simulink model "TP_3tanks_sim"  (R2024b)
settings: Solver=FixedStepAuto  StartTime=0.0  StopTime=100  RelTol=1e-3
values from neighbouring files (symbols this model uses):
  g = 9.8    [inverted_script.m]    (also in tanks_variable.m = 9.82)
  k1 = 0.32    [tanks_variable.m]
  k2 = 0.24    [tanks_variable.m]
  mu13 = 3.21    [tanks_variable.m]
  mu20 = 3.21    [tanks_variable.m]
  mu32 = 3.21    [tanks_variable.m]
  S1 = 0.04    [tanks_variable.m]
  S2 = 0.037    [tanks_variable.m]
  S3 = 0.049    [tanks_variable.m]
  Sp = 4e-4    (= 0.0004)    [tanks_variable.m]
libraries: slpidlib x2
settings Model: Creator=thomas  LastModifiedBy=thomas
settings OptimizationCC: DefaultParameterBehavior=Inlined  EnhancedBackFolding=on  PassReuseOutputArgsAs=Individual arguments  ZeroExternalMemoryAtStartup=off  ZeroInternalMemoryAtStartup=off  MaxStackSize=64  OptimizeBlockOrder=speed  DifferentSizesBufferReuse=on  OptimizationCustomize=off  EfficientTunableParamExpr=on
settings DebuggingCC: ParameterTunabilityLossMsg=error
settings HardwareCC: ProdBitPerLong=64  ProdHWDeviceType=Intel->x86-64 (Linux 64)  UseEmbeddedCoderFeatures=off
settings SFSimCC: MATLABDynamicMemAlloc=off
settings RTWCC: Description=Embedded Coder  SystemTargetFile=ert.tlc  HardwareBoard=Robot Operating System 2 (ROS 2)  TLCOptions="-aInlineSetEventsForThisBaseRateFcn=TLC_FALSE -aSuppressMultiTaskScheduler=TLC_FALSE  -aRateBasedStepFcn=0"  TemplateMakefile=ert_default_tmf  Toolchain=Colcon Tools  TargetLang=C++
settings CodeAppCC: ForceParamTrailComments=on  IgnoreCustomStorageClasses=off  OperatorAnnotations=on  SimulinkDataObjDesc=on  SFDataObjDesc=on  InsertBlockDesc=on
settings ERTTargetCC: CodeInterfacePackaging=C++ class  SupportNonInlinedSFcns=on  RootIOFormat=Structure reference

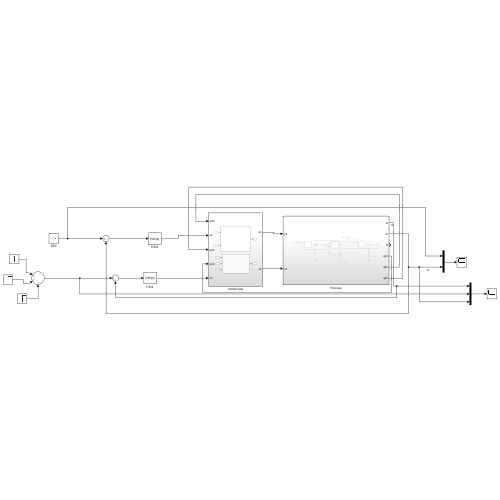
[thumbnail: Simulink's stored preview of the top-level diagram]
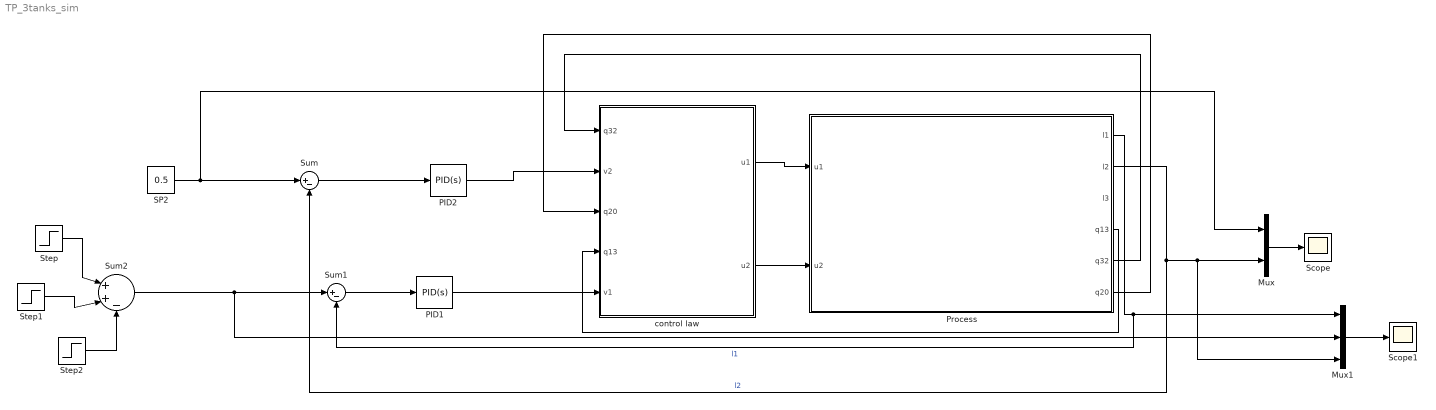
== system TP_3tanks_sim ==
  Mux : Mux  Inputs=2
  Mux1 : Mux  Inputs=3
  PID1 : slpidlib/PID Controller  Controller=PID  Form=Parallel  TimeDomain=Continuous-time  UseExternalTs=off  SampleTime=-1  IntegratorMethod=Forward Euler  FilterMethod=Forward Euler  ControllerParametersSource=internal  P=1  I=1  UseKiTs=off  D=0  UseExternalDerivativeSource=off  N=100  UseFilter=on  TunerSelectOption=Transfer Function Based (PID Tuner App)  InitialConditionSource=internal  InitialConditionForIntegrator=0  InitialConditionForFilter=0  DifferentiatorICPrevScaledInput=0  ExternalReset=none  TrackingMode=off  Kt=1  LimitOutput=off  SatLimitsSource=internal  UpperSaturationLimit=inf  LowerSaturationLimit=-inf  LinearizeAsGain=on  AntiWindupMode=none  Kb=1  LimitIntegrator=off  UpperIntegratorSaturationLimit=inf  LowerIntegratorSaturationLimit=-inf  POutMin=[]  POutMax=[]  IOutMin=[]  IOutMax=[]  DOutMin=[]  DOutMax=[]  NOutMin=[]  NOutMax=[]  SumOutMin=[]  SumOutMax=[]  SaturationOutMin=[]  SaturationOutMax=[]  PParamMin=[]  PParamMax=[]  IParamMin=[]  IParamMax=[]  DParamMin=[]  DParamMax=[]  NParamMin=[]  NParamMax=[]  KbParamMin=[]  KbParamMax=[]  KtParamMin=[]  KtParamMax=[]  KbOutMin=[]  KbOutMax=[]  KtOutMin=[]  KtOutMax=[]  IntegratorOutMin=[]  IntegratorOutMax=[]  FilterOutMin=[]  FilterOutMax=[]  SumI1OutMin=[]  SumI1OutMax=[]  SumI2OutMin=[]  SumI2OutMax=[]  SumI3OutMin=[]  SumI3OutMax=[]  SumI4OutMin=[]  SumI4OutMax=[]  SumDOutMin=[]  SumDOutMax=[]  DifferentiatorOutMin=[]  DifferentiatorOutMax=[]  FilterDiffOutCoefMin=[]  FilterDiffOutCoefMax=[]  ReciprocalOutMin=[]  ReciprocalOutMax=[]  SumDenOutMin=[]  SumDenOutMax=[]  SumNumOutMin=[]  SumNumOutMax=[]  DivideOutMin=[]  DivideOutMax=[]  UdiffTsProdOutMin=[]  UdiffTsProdOutMax=[]  NTsProdOutMin=[]  NTsProdOutMax=[]  UintegralTsProdOutMin=[]  UintegralTsProdOutMax=[]  UngainTsProdOutMin=[]  UngainTsProdOutMax=[]  ClampingZeroOutDataTypeStr=Inherit: Inherit via back propagation  ClampingZeroOutMin=[]  ClampingZeroOutMax=[]  FilterDenConstantOutDataTypeStr=Inherit: Inherit via back propagation  FilterDenConstantOutMin=[]  FilterDenConstantOutMax=[]  PCopyOutDataTypeStr=Inherit: Inherit via back propagation  PCopyOutMin=[]  PCopyOutMax=[]  NCopyOutDataTypeStr=Inherit: Inherit via back propagation  NCopyOutMin=[]  NCopyOutMax=[]  IntegratorContinuousStateAttributes=''  IntegratorStateMustResolveToSignalObject=off  IntegratorRTWStateStorageClass=Auto  FilterContinuousStateAttributes=''  FilterStateMustResolveToSignalObject=off  FilterRTWStateStorageClass=Auto  ParallelPVariant=InternalParameters  IdealPVariant=Disabled  IVariant=InternalParameters  DVariant=InternalParameters  IntegratorVariant=Continuous  SatVariant=Disabled  AWVariant=Passthrough  PCopyVariant=Disabled  TRVariant=Disabled  FdbkBlocksVariant=Forward  IdealPFdbkVariant=Disabled  SatFdbkVariant=Disabled  DerivativeFilterVariant=ContFilter  NVariant=InternalParameters  NCopyVariant=Disabled  FilterICVariant=InternalICsFilter  IntegratorICVariant=InternalICs  ExternalResetVariant=Disabled  TRSumVariant=Passthrough  SumFdbkVariant=Disabled  SumVariant=Sum_PID  TsampFilterVariant=InternalTs  TsampNgainVariant=Passthrough  TsampIntegralVariant=Disabled_SignalSpec  ExternalSaturationOutDataTypeStr=Inherit: Same as second input  DerivativeSourceVariant=ErrorSignal  PreIntVariant=InternalPreInt
  PID2 : slpidlib/PID Controller  Controller=PID  Form=Parallel  TimeDomain=Continuous-time  UseExternalTs=off  SampleTime=-1  IntegratorMethod=Forward Euler  FilterMethod=Forward Euler  ControllerParametersSource=internal  P=1  I=1  UseKiTs=off  D=0  UseExternalDerivativeSource=off  N=100  UseFilter=on  TunerSelectOption=Transfer Function Based (PID Tuner App)  InitialConditionSource=internal  InitialConditionForIntegrator=0  InitialConditionForFilter=0  DifferentiatorICPrevScaledInput=0  ExternalReset=none  TrackingMode=off  Kt=1  LimitOutput=off  SatLimitsSource=internal  UpperSaturationLimit=inf  LowerSaturationLimit=-inf  LinearizeAsGain=on  AntiWindupMode=none  Kb=1  LimitIntegrator=off  UpperIntegratorSaturationLimit=inf  LowerIntegratorSaturationLimit=-inf  POutMin=[]  POutMax=[]  IOutMin=[]  IOutMax=[]  DOutMin=[]  DOutMax=[]  NOutMin=[]  NOutMax=[]  SumOutMin=[]  SumOutMax=[]  SaturationOutMin=[]  SaturationOutMax=[]  PParamMin=[]  PParamMax=[]  IParamMin=[]  IParamMax=[]  DParamMin=[]  DParamMax=[]  NParamMin=[]  NParamMax=[]  KbParamMin=[]  KbParamMax=[]  KtParamMin=[]  KtParamMax=[]  KbOutMin=[]  KbOutMax=[]  KtOutMin=[]  KtOutMax=[]  IntegratorOutMin=[]  IntegratorOutMax=[]  FilterOutMin=[]  FilterOutMax=[]  SumI1OutMin=[]  SumI1OutMax=[]  SumI2OutMin=[]  SumI2OutMax=[]  SumI3OutMin=[]  SumI3OutMax=[]  SumI4OutMin=[]  SumI4OutMax=[]  SumDOutMin=[]  SumDOutMax=[]  DifferentiatorOutMin=[]  DifferentiatorOutMax=[]  FilterDiffOutCoefMin=[]  FilterDiffOutCoefMax=[]  ReciprocalOutMin=[]  ReciprocalOutMax=[]  SumDenOutMin=[]  SumDenOutMax=[]  SumNumOutMin=[]  SumNumOutMax=[]  DivideOutMin=[]  DivideOutMax=[]  UdiffTsProdOutMin=[]  UdiffTsProdOutMax=[]  NTsProdOutMin=[]  NTsProdOutMax=[]  UintegralTsProdOutMin=[]  UintegralTsProdOutMax=[]  UngainTsProdOutMin=[]  UngainTsProdOutMax=[]  ClampingZeroOutDataTypeStr=Inherit: Inherit via back propagation  ClampingZeroOutMin=[]  ClampingZeroOutMax=[]  FilterDenConstantOutDataTypeStr=Inherit: Inherit via back propagation  FilterDenConstantOutMin=[]  FilterDenConstantOutMax=[]  PCopyOutDataTypeStr=Inherit: Inherit via back propagation  PCopyOutMin=[]  PCopyOutMax=[]  NCopyOutDataTypeStr=Inherit: Inherit via back propagation  NCopyOutMin=[]  NCopyOutMax=[]  IntegratorContinuousStateAttributes=''  IntegratorStateMustResolveToSignalObject=off  IntegratorRTWStateStorageClass=Auto  FilterContinuousStateAttributes=''  FilterStateMustResolveToSignalObject=off  FilterRTWStateStorageClass=Auto  ParallelPVariant=InternalParameters  IdealPVariant=Disabled  IVariant=InternalParameters  DVariant=InternalParameters  IntegratorVariant=Continuous  SatVariant=Disabled  AWVariant=Passthrough  PCopyVariant=Disabled  TRVariant=Disabled  FdbkBlocksVariant=Forward  IdealPFdbkVariant=Disabled  SatFdbkVariant=Disabled  DerivativeFilterVariant=ContFilter  NVariant=InternalParameters  NCopyVariant=Disabled  FilterICVariant=InternalICsFilter  IntegratorICVariant=InternalICs  ExternalResetVariant=Disabled  TRSumVariant=Passthrough  SumFdbkVariant=Disabled  SumVariant=Sum_PID  TsampFilterVariant=InternalTs  TsampNgainVariant=Passthrough  TsampIntegralVariant=Disabled_SignalSpec  ExternalSaturationOutDataTypeStr=Inherit: Same as second input  DerivativeSourceVariant=ErrorSignal  PreIntVariant=InternalPreInt
  Process : Subsystem
  SP2 : Constant  Value=0.5
  Scope : Scope
  Scope1 : Scope
  Step : Step  Time=30  After=0.4  SampleTime=0.001
  Step1 : Step  Time=60  After=0.3  SampleTime=0
  Step2 : Step  Time=90  After=0.45  SampleTime=0
  Sum : Sum  Inputs=|+-
  Sum1 : Sum  Inputs=|+-
  Sum2 : Sum  Inputs=|++-
  control law : Subsystem
  wires:
  Mux/1 -> Scope/1
  Process/2(l2) -> Mux1/3, Mux/2, Sum/2  "l2"
  Process/1(l1) -> Sum1/2, Mux1/1  "l1"
  Process/6(q20) -> control law/3(q20)
  Process/5(q32) -> control law/1(q32)
  Process/4(q13) -> control law/4(q13)
  PID1/1 -> control law/5(v1)
  Sum/1 -> PID2/1
  Sum1/1 -> PID1/1
  PID2/1 -> control law/2(v2)
  SP2/1 -> Mux/1, Sum/1
  Sum2/1 -> Mux1/2, Sum1/1
  control law/1(u1) -> Process/1(u1)
  control law/2(u2) -> Process/2(u2)
  Mux1/1 -> Scope1/1
  Step/1 -> Sum2/1
  Step1/1 -> Sum2/2
  Step2/1 -> Sum2/3

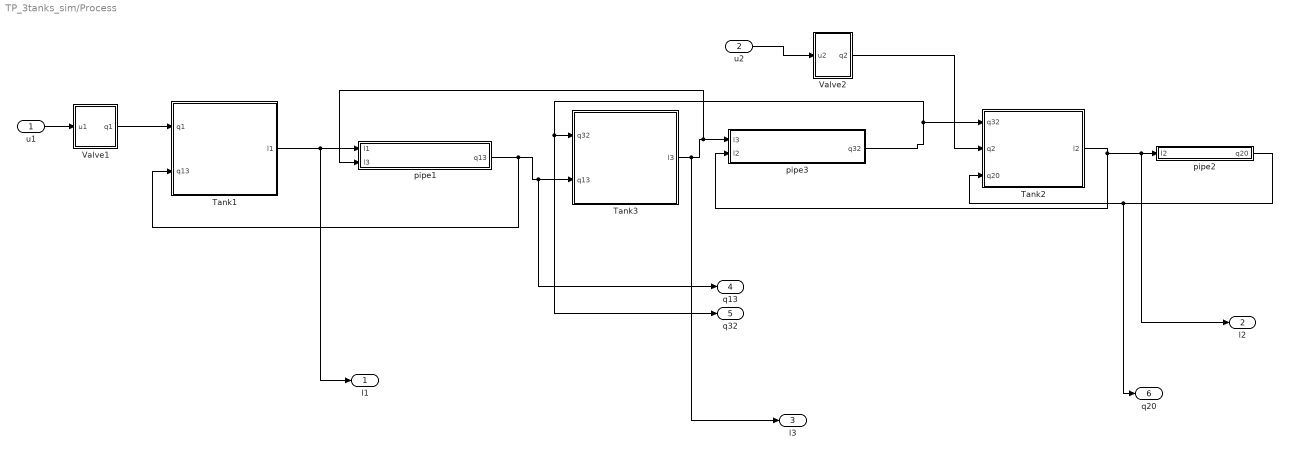
== system TP_3tanks_sim/Process ==
  u1 : Inport
  u2 : Inport  Port=2
  Tank1 : Subsystem
  Tank2 : Subsystem
  Tank3 : Subsystem
  Valve1 : Subsystem
  Valve2 : Subsystem
  pipe1 : Subsystem
  pipe2 : Subsystem
  pipe3 : Subsystem
  l1 : Outport
  l2 : Outport  Port=2
  l3 : Outport  Port=3
  q13 : Outport  Port=4
  q32 : Outport  Port=5
  q20 : Outport  Port=6
  wires:
  Valve1/1(q1) -> Tank1/1(q1)
  u1/1 -> Valve1/1(u1)
  pipe3/1(q32) -> q32/1, Tank3/1(q32), Tank2/1(q32)
  Tank2/1(l2) -> pipe3/2(l2), l2/1, pipe2/1(l2)
  Valve2/1(q2) -> Tank2/2(q2)
  pipe1/1(q13) -> Tank1/2(q13), q13/1, Tank3/2(q13)
  Tank3/1(l3) -> l3/1, pipe1/2(l3), pipe3/1(l3)
  u2/1 -> Valve2/1(u2)
  Tank1/1(l1) -> l1/1, pipe1/1(l1)
  pipe2/1(q20) -> q20/1, Tank2/3(q20)

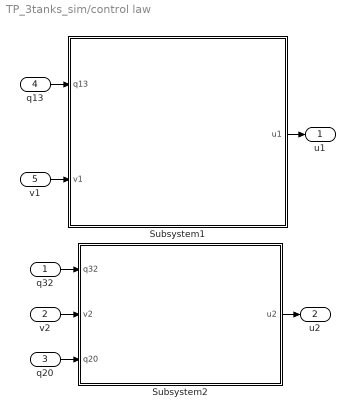
== system TP_3tanks_sim/control law ==
  q32 : Inport
  v2 : Inport  Port=2
  q20 : Inport  Port=3
  q13 : Inport  Port=4
  v1 : Inport  Port=5
  Subsystem1 : Subsystem
  Subsystem2 : Subsystem
  u1 : Outport
  u2 : Outport  Port=2
  wires:
  q13/1 -> Subsystem1/1(q13)
  v2/1 -> Subsystem2/2(v2)
  Subsystem2/1(u2) -> u2/1
  q20/1 -> Subsystem2/3(q20)
  q32/1 -> Subsystem2/1(q32)
  Subsystem1/1(u1) -> u1/1
  v1/1 -> Subsystem1/2(v1)

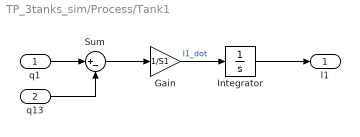
== system TP_3tanks_sim/Process/Tank1 ==
  q1 : Inport
  q13 : Inport  Port=2
  Gain : Gain  Gain=1/S1
  Integrator : Integrator
  Sum : Sum  Inputs=|+-
  l1 : Outport
  wires:
  q1/1 -> Sum/1
  Gain/1 -> Integrator/1  "l1_dot"
  Sum/1 -> Gain/1
  Integrator/1 -> l1/1
  q13/1 -> Sum/2

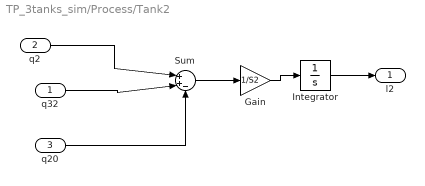
== system TP_3tanks_sim/Process/Tank2 ==
  q32 : Inport
  q2 : Inport  Port=2
  q20 : Inport  Port=3
  Gain : Gain  Gain=1/S2
  Integrator : Integrator
  Sum : Sum  Inputs=|++-
  l2 : Outport
  wires:
  Gain/1 -> Integrator/1
  Integrator/1 -> l2/1
  Sum/1 -> Gain/1
  q32/1 -> Sum/2
  q20/1 -> Sum/3
  q2/1 -> Sum/1

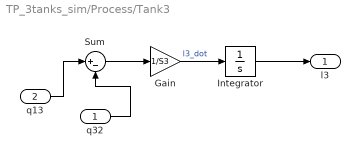
== system TP_3tanks_sim/Process/Tank3 ==
  q32 : Inport
  q13 : Inport  Port=2
  Gain : Gain  Gain=1/S3
  Integrator : Integrator
  Sum : Sum  Inputs=|+-
  l3 : Outport
  wires:
  q13/1 -> Sum/1
  Integrator/1 -> l3/1
  Sum/1 -> Gain/1
  Gain/1 -> Integrator/1  "l3_dot"
  q32/1 -> Sum/2

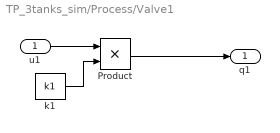
== system TP_3tanks_sim/Process/Valve1 ==
  u1 : Inport
  Product : Product
  k1 : Constant  Value=k1
  q1 : Outport
  wires:
  Product/1 -> q1/1
  u1/1 -> Product/1
  k1/1 -> Product/2

== system TP_3tanks_sim/Process/Valve2 ==
  u2 : Inport
  Product : Product
  k2 : Constant  Value=k2
  q2 : Outport
  wires:
  k2/1 -> Product/2
  u2/1 -> Product/1
  Product/1 -> q2/1

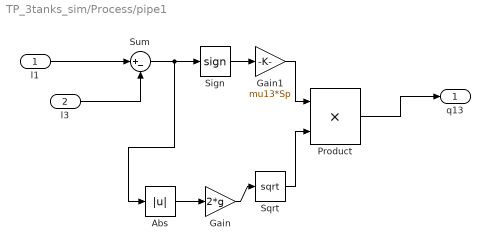
== system TP_3tanks_sim/Process/pipe1 ==
  l1 : Inport
  l3 : Inport  Port=2
  Abs : Abs  SaturateOnIntegerOverflow=off
  Gain : Gain  Gain=2*g
  Gain1 : Gain  Gain=mu13*Sp
  Product : Product
  Sign : Signum
  Sqrt : Sqrt
  Sum : Sum  Inputs=|+-
  q13 : Outport
  wires:
  l1/1 -> Sum/1
  Sign/1 -> Gain1/1
  Sqrt/1 -> Product/2
  Sum/1 -> Abs/1, Sign/1
  Gain1/1 -> Product/1
  Abs/1 -> Gain/1
  Gain/1 -> Sqrt/1
  l3/1 -> Sum/2
  Product/1 -> q13/1

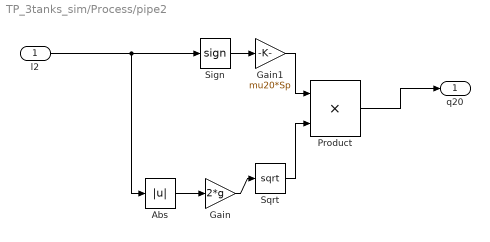
== system TP_3tanks_sim/Process/pipe2 ==
  l2 : Inport
  Abs : Abs  SaturateOnIntegerOverflow=off
  Gain : Gain  Gain=2*g
  Gain1 : Gain  Gain=mu20*Sp
  Product : Product
  Sign : Signum
  Sqrt : Sqrt
  q20 : Outport
  wires:
  Sign/1 -> Gain1/1
  Sqrt/1 -> Product/2
  Gain1/1 -> Product/1
  Abs/1 -> Gain/1
  Gain/1 -> Sqrt/1
  Product/1 -> q20/1
  l2/1 -> Abs/1, Sign/1

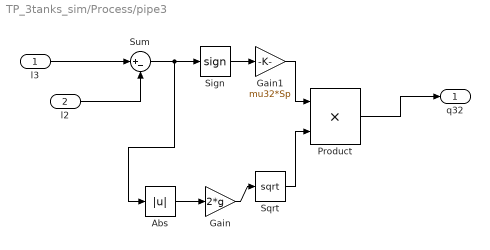
== system TP_3tanks_sim/Process/pipe3 ==
  l3 : Inport
  l2 : Inport  Port=2
  Abs : Abs  SaturateOnIntegerOverflow=off
  Gain : Gain  Gain=2*g
  Gain1 : Gain  Gain=mu32*Sp
  Product : Product
  Sign : Signum
  Sqrt : Sqrt
  Sum : Sum  Inputs=|+-
  q32 : Outport
  wires:
  l3/1 -> Sum/1
  Sign/1 -> Gain1/1
  Sqrt/1 -> Product/2
  Sum/1 -> Abs/1, Sign/1
  Gain1/1 -> Product/1
  Abs/1 -> Gain/1
  Gain/1 -> Sqrt/1
  l2/1 -> Sum/2
  Product/1 -> q32/1

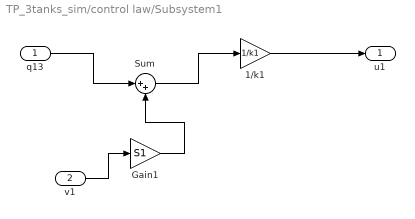
== system TP_3tanks_sim/control law/Subsystem1 ==
  q13 : Inport
  v1 : Inport  Port=2
  1/k1 : Gain  Gain=1/k1
  Gain1 : Gain  Gain=S1
  Sum : Sum  Inputs=|++
  u1 : Outport
  wires:
  q13/1 -> Sum/1
  v1/1 -> Gain1/1
  Sum/1 -> 1/k1/1
  1/k1/1 -> u1/1
  Gain1/1 -> Sum/2

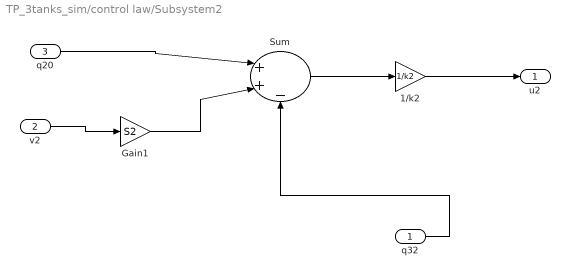
== system TP_3tanks_sim/control law/Subsystem2 ==
  q32 : Inport
  v2 : Inport  Port=2
  q20 : Inport  Port=3
  1/k2 : Gain  Gain=1/k2
  Gain1 : Gain  Gain=S2
  Sum : Sum  Inputs=|++-
  u2 : Outport
  wires:
  q32/1 -> Sum/3
  v2/1 -> Gain1/1
  Sum/1 -> 1/k2/1
  1/k2/1 -> u2/1
  Gain1/1 -> Sum/2
  q20/1 -> Sum/1
